simulink model "Q4"  (R2020b)
settings: Solver=VariableStepAuto  StartTime=0.0  StopTime=10.0  RelTol=1e-3
settings Model: Creator=Javad  LastModifiedBy=Javad
settings SolverCC: ZeroCrossAlgorithm=Adaptive
settings DebuggingCC: IgnoredZcDiagnostic=none

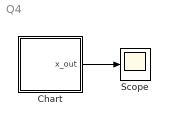
== system Q4 ==
  Chart : Stateflow chart  TreatAsAtomicUnit=on
  Scope : Scope
  wires:
  Chart/1(x_out) -> Scope/1

== stateflow chart Q4/Chart ==
  settings: updateMethod=CONTINUOUS
  state q1
    du:
    x_dot=1;
    x_out=x;
  state q2
    du:
    x_dot=-1;
    x_out=x;
  (default) -> q1 : {x=-1;}
  q1 -> q2 [order 1] : [x>=0]{x=x;}
  q1 -> q1 [order 2] : [x<=-3]{x=x;}
  data: x_out output; x local
  data x settings: updateMethod=SF_CONTINUOUS_TIME_DATA
